simulink model "frequency_only"  (R2012b)
settings: Solver=ode45  StartTime=0.0  StopTime=41000*512  RelTol=1e-3
libraries: xbsIndex_r4 x14823, casper_library_misc x115, casper_library_multipliers x20, casper_library_delays x13, simulink x3, xps_library x3, dspsrcs4 x2, xbsReplacements_r4 x2
(part 5 of 146)

== system frequency_only/accumulators/accumulator_0x1 ==
  note: Note: in1 = MSB, in2 = LSB
  note: We want out vacc to keep full resolution
  new_acc : Inport
  bus_in : Inport  Port=2
  Convert{,1..3} (4 alike) : xbsIndex_r4/Convert  gui_display_data_type=Fixed-point  arith_type="Signed  (2's comp)"  n_bits=64  bin_pt=34  float_type=Single  exp_bits=8  fraction_bits=24  quantization=Truncate  overflow=Wrap  en=off  latency=0  dbl_ovrd=off  pipeline=off  block_type=convert
  Delay{,1..4} (5 alike) : xbsIndex_r4/Delay  rst=off  infoeditControl=Selection of Reset will increase slice count due to use of real FFs and instead of SRLs  en=off  latency=1  dbl_ovrd=off  reg_retiming=off  block_type=delay
  Logical : xbsIndex_r4/Logical  logical_function=OR  inputs=4  en=off  latency=1  precision=Full  arith_type=Unsigned  n_bits=16  bin_pt=0  align_bp=on  dbl_ovrd=off  block_type=logical
  Terminator : Terminator
  Terminator1 : Terminator
  Terminator2 : Terminator
  bus_create1 : Subsystem  AncestorBlock=casper_library_flow_control/bus_create  mask(bus_create){inputNum=2}
      mask prompts: inputNum "Number of inputs:"
      mask init:
      | bus_create_init(gcb,...
      |     'inputNum', inputNum);
  bus_create2 : Subsystem  AncestorBlock=casper_library_flow_control/bus_create  mask(bus_create){inputNum=2}
      mask prompts: inputNum "Number of inputs:"
      mask init:
      | bus_create_init(gcb,...
      |     'inputNum', inputNum);
  bus_create4 : Subsystem  AncestorBlock=casper_library_flow_control/bus_create  mask(bus_create){inputNum=2}
      mask prompts: inputNum "Number of inputs:"
      mask init:
      | bus_create_init(gcb,...
      |     'inputNum', inputNum);
  bus_expand : Subsystem  AncestorBlock=casper_library_flow_control/bus_expand  mask(bus_expand){mode=divisions of equal size, outputNum=2, outputWidth=bitwidth_in*2, outputBinaryPt=0, outputArithmeticType=0, show_format=off, outputToWorkspace=off, variablePrefix=out, outputToModelAsWell=on}
      mask prompts: outputNum "Number of outputs:"; outputWidth "Output width:"; outputBinaryPt "Output binary point position:"; outputArithmeticType "Output arithmetic type (ufix=0, fix=1, bool=2):"; show_format "Print format string?"; outputToWorkspace "Output to workspace?"; variablePrefix "Variable name prefix:"; outputToModelAsWell "Output to model as well?"
      mask help:
      | Expands a 'bus' made using a bus_create or Xilinx
      | concat block.
      | The input will be divided into the specified number
      | of outputs with the specified arithmetic types.
      | Divisions are made from most significant bit.
      mask init: same as frequency_only/bus_expand
      settings: AttributesFormatString=2 outputs
      mask TypeOptions mode: divisions of equal size | divisions of arbitrary size
      mask Callback mode: bus_expand_callback();
      mask Callback outputWidth: bus_expand_callback();
      mask Callback outputToWorkspace: bus_expand_callback();
  dsp48e_bram_vacc_lsb_im : Subsystem  AncestorBlock=casper_library_accumulators/dsp48e_bram_vacc  mask(dsp48e_bram_vacc){vec_len=vector_length, arith_type=Signed  (2's comp), bin_pt_in=bin_point_in, n_bits_out=bitwidth_out, convert_latency=1}
      mask prompts: vec_len "Vector length:"; arith_type "Output type:"; bin_pt_in "Binary point (input):"; n_bits_out "Bit width (output):"; convert_latency "Convert Latency"
      mask help:
      | A vector accumulator modeled after a shift register.  It outputs its previous accumulated vector after a new_acc pulse is received.
      |
      | Based on the simple_bram_vacc block, this version replaces the adder and mux with a single DSP48E block, allowing high-speed compilation.
      |
      | The input and outputs ports are limited to 48 bits. Overflow is indicated with a line out.
      |
      | Each accumulation uses the full 48 bits, irrespective of mask parameters.
      | The output of the accumulation then slices off the output bits.
      | The binary point is kept at the same relative location to ensure that the signal value is not changed.
      mask init:
      | dsp48e_bram_vacc_init(gcb, ...
      |     'vec_len', vec_len, ...
      |     'arith_type', arith_type, ...
      |     'bin_pt_in', bin_pt_in, ...
      |     'n_bits_out', n_bits_out, ...
      |     'convert_latency', convert_latency);
      mask TypeOptions arith_type: Unsigned | Signed  (2's comp)
  dsp48e_bram_vacc_lsb_re : Subsystem  AncestorBlock=casper_library_accumulators/dsp48e_bram_vacc  mask(dsp48e_bram_vacc){vec_len=vector_length, arith_type=Signed  (2's comp), bin_pt_in=bin_point_in, n_bits_out=bitwidth_out, convert_latency=1}
      mask prompts: vec_len "Vector length:"; arith_type "Output type:"; bin_pt_in "Binary point (input):"; n_bits_out "Bit width (output):"; convert_latency "Convert Latency"
      mask help:
      | A vector accumulator modeled after a shift register.  It outputs its previous accumulated vector after a new_acc pulse is received.
      |
      | Based on the simple_bram_vacc block, this version replaces the adder and mux with a single DSP48E block, allowing high-speed compilation.
      |
      | The input and outputs ports are limited to 48 bits. Overflow is indicated with a line out.
      |
      | Each accumulation uses the full 48 bits, irrespective of mask parameters.
      | The output of the accumulation then slices off the output bits.
      | The binary point is kept at the same relative location to ensure that the signal value is not changed.
      mask init:
      | dsp48e_bram_vacc_init(gcb, ...
      |     'vec_len', vec_len, ...
      |     'arith_type', arith_type, ...
      |     'bin_pt_in', bin_pt_in, ...
      |     'n_bits_out', n_bits_out, ...
      |     'convert_latency', convert_latency);
      mask TypeOptions arith_type: Unsigned | Signed  (2's comp)
  dsp48e_bram_vacc_msb_im : Subsystem  AncestorBlock=casper_library_accumulators/dsp48e_bram_vacc  mask(dsp48e_bram_vacc){vec_len=vector_length, arith_type=Signed  (2's comp), bin_pt_in=bin_point_in, n_bits_out=bitwidth_out, convert_latency=1}
      mask prompts: vec_len "Vector length:"; arith_type "Output type:"; bin_pt_in "Binary point (input):"; n_bits_out "Bit width (output):"; convert_latency "Convert Latency"
      mask help:
      | A vector accumulator modeled after a shift register.  It outputs its previous accumulated vector after a new_acc pulse is received.
      |
      | Based on the simple_bram_vacc block, this version replaces the adder and mux with a single DSP48E block, allowing high-speed compilation.
      |
      | The input and outputs ports are limited to 48 bits. Overflow is indicated with a line out.
      |
      | Each accumulation uses the full 48 bits, irrespective of mask parameters.
      | The output of the accumulation then slices off the output bits.
      | The binary point is kept at the same relative location to ensure that the signal value is not changed.
      mask init:
      | dsp48e_bram_vacc_init(gcb, ...
      |     'vec_len', vec_len, ...
      |     'arith_type', arith_type, ...
      |     'bin_pt_in', bin_pt_in, ...
      |     'n_bits_out', n_bits_out, ...
      |     'convert_latency', convert_latency);
      mask TypeOptions arith_type: Unsigned | Signed  (2's comp)
  dsp48e_bram_vacc_msb_re : Subsystem  AncestorBlock=casper_library_accumulators/dsp48e_bram_vacc  mask(dsp48e_bram_vacc){vec_len=vector_length, arith_type=Signed  (2's comp), bin_pt_in=bin_point_in, n_bits_out=bitwidth_out, convert_latency=1}
      mask prompts: vec_len "Vector length:"; arith_type "Output type:"; bin_pt_in "Binary point (input):"; n_bits_out "Bit width (output):"; convert_latency "Convert Latency"
      mask help:
      | A vector accumulator modeled after a shift register.  It outputs its previous accumulated vector after a new_acc pulse is received.
      |
      | Based on the simple_bram_vacc block, this version replaces the adder and mux with a single DSP48E block, allowing high-speed compilation.
      |
      | The input and outputs ports are limited to 48 bits. Overflow is indicated with a line out.
      |
      | Each accumulation uses the full 48 bits, irrespective of mask parameters.
      | The output of the accumulation then slices off the output bits.
      | The binary point is kept at the same relative location to ensure that the signal value is not changed.
      mask init:
      | dsp48e_bram_vacc_init(gcb, ...
      |     'vec_len', vec_len, ...
      |     'arith_type', arith_type, ...
      |     'bin_pt_in', bin_pt_in, ...
      |     'n_bits_out', n_bits_out, ...
      |     'convert_latency', convert_latency);
      mask TypeOptions arith_type: Unsigned | Signed  (2's comp)
  lsb_c_to_ri : casper_library_misc/c_to_ri  n_bits=bitwidth_in  bin_pt=bin_point_in
      settings: AttributesFormatString=37_34 r/i
  msb_c_to_ri : casper_library_misc/c_to_ri  n_bits=bitwidth_in  bin_pt=bin_point_in
      settings: AttributesFormatString=37_34 r/i
  acc_valid : Outport
  bus_out : Outport  Port=2
  carry : Outport  Port=3
  wires:
  Logical/1 -> carry/1
  [c_lsb_im] -> Logical/4
  [c_lsb_re] -> Logical/3
  [c_msb_im] -> Logical/2
  [c_msb_re] -> Logical/1
  dsp48e_bram_vacc_lsb_im/3(carry) -> [c_lsb_im]
  dsp48e_bram_vacc_lsb_im/1(dout) -> Convert3/1
  dsp48e_bram_vacc_lsb_re/3(carry) -> [c_lsb_re]
  dsp48e_bram_vacc_msb_im/3(carry) -> [c_msb_im]
  dsp48e_bram_vacc_msb_re/3(carry) -> [c_msb_re]
  Convert3/1 -> bus_create1/2(in2)
  Convert2/1 -> bus_create1/1(in1)
  Convert1/1 -> bus_create4/2(in2)
  Convert/1 -> bus_create4/1(in1)
  Delay4/1 -> dsp48e_bram_vacc_lsb_im/2(din)
  Delay3/1 -> dsp48e_bram_vacc_lsb_re/2(din)
  Delay2/1 -> dsp48e_bram_vacc_msb_im/2(din)
  Delay1/1 -> dsp48e_bram_vacc_msb_re/2(din)
  Delay/1 -> [new_acc]
  [new_acc] -> dsp48e_bram_vacc_msb_re/1(new_acc)
  lsb_c_to_ri/2 -> Delay4/1
  lsb_c_to_ri/1 -> Delay3/1
  msb_c_to_ri/2 -> Delay2/1
  msb_c_to_ri/1 -> Delay1/1
  bus_in/1 -> bus_expand/1(bus_in)
  bus_create2/1(bus_out) -> bus_out/1
  dsp48e_bram_vacc_msb_re/1(dout) -> Convert/1
  dsp48e_bram_vacc_msb_im/1(dout) -> Convert1/1
  dsp48e_bram_vacc_lsb_re/1(dout) -> Convert2/1
  new_acc/1 -> Delay/1
  bus_create1/1(bus_out) -> bus_create2/2(in2)
  bus_create4/1(bus_out) -> bus_create2/1(in1)
  [new_acc] -> dsp48e_bram_vacc_lsb_im/1(new_acc)
  [new_acc] -> dsp48e_bram_vacc_lsb_re/1(new_acc)
  [new_acc] -> dsp48e_bram_vacc_msb_im/1(new_acc)
  dsp48e_bram_vacc_msb_re/2(valid) -> acc_valid/1
  bus_expand/2(lsb_out1) -> lsb_c_to_ri/1
  bus_expand/1(msb_out2) -> msb_c_to_ri/1
  dsp48e_bram_vacc_lsb_re/2(valid) -> Terminator1/1
  dsp48e_bram_vacc_msb_im/2(valid) -> Terminator/1
  dsp48e_bram_vacc_lsb_im/2(valid) -> Terminator2/1

== system frequency_only/accumulators/accumulator_0x2 ==
  note: We want out vacc to keep full resolution
  note: Note: in1 = MSB, in2 = LSB
  new_acc : Inport
  bus_in : Inport  Port=2
  Convert{,1..3} (4 alike) : xbsIndex_r4/Convert  gui_display_data_type=Fixed-point  arith_type="Signed  (2's comp)"  n_bits=64  bin_pt=34  float_type=Single  exp_bits=8  fraction_bits=24  quantization=Truncate  overflow=Wrap  en=off  latency=0  dbl_ovrd=off  pipeline=off  block_type=convert
  Delay{,1..4} (5 alike) : xbsIndex_r4/Delay  rst=off  infoeditControl=Selection of Reset will increase slice count due to use of real FFs and instead of SRLs  en=off  latency=1  dbl_ovrd=off  reg_retiming=off  block_type=delay
  Logical : xbsIndex_r4/Logical  logical_function=OR  inputs=4  en=off  latency=1  precision=Full  arith_type=Unsigned  n_bits=16  bin_pt=0  align_bp=on  dbl_ovrd=off  block_type=logical
  Terminator : Terminator
  Terminator1 : Terminator
  Terminator2 : Terminator
  bus_create1 : Subsystem  AncestorBlock=casper_library_flow_control/bus_create  mask(bus_create){inputNum=2}
      mask prompts: inputNum "Number of inputs:"
      mask init:
      | bus_create_init(gcb,...
      |     'inputNum', inputNum);
  bus_create2 : Subsystem  AncestorBlock=casper_library_flow_control/bus_create  mask(bus_create){inputNum=2}
      mask prompts: inputNum "Number of inputs:"
      mask init:
      | bus_create_init(gcb,...
      |     'inputNum', inputNum);
  bus_create4 : Subsystem  AncestorBlock=casper_library_flow_control/bus_create  mask(bus_create){inputNum=2}
      mask prompts: inputNum "Number of inputs:"
      mask init:
      | bus_create_init(gcb,...
      |     'inputNum', inputNum);
  bus_expand : Subsystem  AncestorBlock=casper_library_flow_control/bus_expand  mask(bus_expand){mode=divisions of equal size, outputNum=2, outputWidth=bitwidth_in*2, outputBinaryPt=0, outputArithmeticType=0, show_format=off, outputToWorkspace=off, variablePrefix=out, outputToModelAsWell=on}
      mask prompts: outputNum "Number of outputs:"; outputWidth "Output width:"; outputBinaryPt "Output binary point position:"; outputArithmeticType "Output arithmetic type (ufix=0, fix=1, bool=2):"; show_format "Print format string?"; outputToWorkspace "Output to workspace?"; variablePrefix "Variable name prefix:"; outputToModelAsWell "Output to model as well?"
      mask help:
      | Expands a 'bus' made using a bus_create or Xilinx
      | concat block.
      | The input will be divided into the specified number
      | of outputs with the specified arithmetic types.
      | Divisions are made from most significant bit.
      mask init: same as frequency_only/bus_expand
      settings: AttributesFormatString=2 outputs
      mask TypeOptions mode: divisions of equal size | divisions of arbitrary size
      mask Callback mode: bus_expand_callback();
      mask Callback outputWidth: bus_expand_callback();
      mask Callback outputToWorkspace: bus_expand_callback();
  dsp48e_bram_vacc_lsb_im : Subsystem  AncestorBlock=casper_library_accumulators/dsp48e_bram_vacc  mask(dsp48e_bram_vacc){vec_len=vector_length, arith_type=Signed  (2's comp), bin_pt_in=bin_point_in, n_bits_out=bitwidth_out, convert_latency=1}
      mask prompts: vec_len "Vector length:"; arith_type "Output type:"; bin_pt_in "Binary point (input):"; n_bits_out "Bit width (output):"; convert_latency "Convert Latency"
      mask help:
      | A vector accumulator modeled after a shift register.  It outputs its previous accumulated vector after a new_acc pulse is received.
      |
      | Based on the simple_bram_vacc block, this version replaces the adder and mux with a single DSP48E block, allowing high-speed compilation.
      |
      | The input and outputs ports are limited to 48 bits. Overflow is indicated with a line out.
      |
      | Each accumulation uses the full 48 bits, irrespective of mask parameters.
      | The output of the accumulation then slices off the output bits.
      | The binary point is kept at the same relative location to ensure that the signal value is not changed.
      mask init:
      | dsp48e_bram_vacc_init(gcb, ...
      |     'vec_len', vec_len, ...
      |     'arith_type', arith_type, ...
      |     'bin_pt_in', bin_pt_in, ...
      |     'n_bits_out', n_bits_out, ...
      |     'convert_latency', convert_latency);
      mask TypeOptions arith_type: Unsigned | Signed  (2's comp)
  dsp48e_bram_vacc_lsb_re : Subsystem  AncestorBlock=casper_library_accumulators/dsp48e_bram_vacc  mask(dsp48e_bram_vacc){vec_len=vector_length, arith_type=Signed  (2's comp), bin_pt_in=bin_point_in, n_bits_out=bitwidth_out, convert_latency=1}
      mask prompts: vec_len "Vector length:"; arith_type "Output type:"; bin_pt_in "Binary point (input):"; n_bits_out "Bit width (output):"; convert_latency "Convert Latency"
      mask help:
      | A vector accumulator modeled after a shift register.  It outputs its previous accumulated vector after a new_acc pulse is received.
      |
      | Based on the simple_bram_vacc block, this version replaces the adder and mux with a single DSP48E block, allowing high-speed compilation.
      |
      | The input and outputs ports are limited to 48 bits. Overflow is indicated with a line out.
      |
      | Each accumulation uses the full 48 bits, irrespective of mask parameters.
      | The output of the accumulation then slices off the output bits.
      | The binary point is kept at the same relative location to ensure that the signal value is not changed.
      mask init:
      | dsp48e_bram_vacc_init(gcb, ...
      |     'vec_len', vec_len, ...
      |     'arith_type', arith_type, ...
      |     'bin_pt_in', bin_pt_in, ...
      |     'n_bits_out', n_bits_out, ...
      |     'convert_latency', convert_latency);
      mask TypeOptions arith_type: Unsigned | Signed  (2's comp)
  dsp48e_bram_vacc_msb_im : Subsystem  AncestorBlock=casper_library_accumulators/dsp48e_bram_vacc  mask(dsp48e_bram_vacc){vec_len=vector_length, arith_type=Signed  (2's comp), bin_pt_in=bin_point_in, n_bits_out=bitwidth_out, convert_latency=1}
      mask prompts: vec_len "Vector length:"; arith_type "Output type:"; bin_pt_in "Binary point (input):"; n_bits_out "Bit width (output):"; convert_latency "Convert Latency"
      mask help:
      | A vector accumulator modeled after a shift register.  It outputs its previous accumulated vector after a new_acc pulse is received.
      |
      | Based on the simple_bram_vacc block, this version replaces the adder and mux with a single DSP48E block, allowing high-speed compilation.
      |
      | The input and outputs ports are limited to 48 bits. Overflow is indicated with a line out.
      |
      | Each accumulation uses the full 48 bits, irrespective of mask parameters.
      | The output of the accumulation then slices off the output bits.
      | The binary point is kept at the same relative location to ensure that the signal value is not changed.
      mask init:
      | dsp48e_bram_vacc_init(gcb, ...
      |     'vec_len', vec_len, ...
      |     'arith_type', arith_type, ...
      |     'bin_pt_in', bin_pt_in, ...
      |     'n_bits_out', n_bits_out, ...
      |     'convert_latency', convert_latency);
      mask TypeOptions arith_type: Unsigned | Signed  (2's comp)
  dsp48e_bram_vacc_msb_re : Subsystem  AncestorBlock=casper_library_accumulators/dsp48e_bram_vacc  mask(dsp48e_bram_vacc){vec_len=vector_length, arith_type=Signed  (2's comp), bin_pt_in=bin_point_in, n_bits_out=bitwidth_out, convert_latency=1}
      mask prompts: vec_len "Vector length:"; arith_type "Output type:"; bin_pt_in "Binary point (input):"; n_bits_out "Bit width (output):"; convert_latency "Convert Latency"
      mask help:
      | A vector accumulator modeled after a shift register.  It outputs its previous accumulated vector after a new_acc pulse is received.
      |
      | Based on the simple_bram_vacc block, this version replaces the adder and mux with a single DSP48E block, allowing high-speed compilation.
      |
      | The input and outputs ports are limited to 48 bits. Overflow is indicated with a line out.
      |
      | Each accumulation uses the full 48 bits, irrespective of mask parameters.
      | The output of the accumulation then slices off the output bits.
      | The binary point is kept at the same relative location to ensure that the signal value is not changed.
      mask init:
      | dsp48e_bram_vacc_init(gcb, ...
      |     'vec_len', vec_len, ...
      |     'arith_type', arith_type, ...
      |     'bin_pt_in', bin_pt_in, ...
      |     'n_bits_out', n_bits_out, ...
      |     'convert_latency', convert_latency);
      mask TypeOptions arith_type: Unsigned | Signed  (2's comp)
  lsb_c_to_ri : casper_library_misc/c_to_ri  n_bits=bitwidth_in  bin_pt=bin_point_in
      settings: AttributesFormatString=37_34 r/i
  msb_c_to_ri : casper_library_misc/c_to_ri  n_bits=bitwidth_in  bin_pt=bin_point_in
      settings: AttributesFormatString=37_34 r/i
  acc_valid : Outport
  bus_out : Outport  Port=2
  carry : Outport  Port=3
  wires:
  dsp48e_bram_vacc_lsb_im/2(valid) -> Terminator2/1
  dsp48e_bram_vacc_msb_im/2(valid) -> Terminator/1
  dsp48e_bram_vacc_lsb_re/2(valid) -> Terminator1/1
  bus_expand/1(msb_out2) -> msb_c_to_ri/1
  bus_expand/2(lsb_out1) -> lsb_c_to_ri/1
  dsp48e_bram_vacc_msb_re/2(valid) -> acc_valid/1
  [new_acc] -> dsp48e_bram_vacc_msb_im/1(new_acc)
  [new_acc] -> dsp48e_bram_vacc_lsb_re/1(new_acc)
  [new_acc] -> dsp48e_bram_vacc_lsb_im/1(new_acc)
  bus_create4/1(bus_out) -> bus_create2/1(in1)
  bus_create1/1(bus_out) -> bus_create2/2(in2)
  new_acc/1 -> Delay/1
  dsp48e_bram_vacc_lsb_re/1(dout) -> Convert2/1
  dsp48e_bram_vacc_msb_im/1(dout) -> Convert1/1
  dsp48e_bram_vacc_msb_re/1(dout) -> Convert/1
  bus_create2/1(bus_out) -> bus_out/1
  bus_in/1 -> bus_expand/1(bus_in)
  msb_c_to_ri/1 -> Delay1/1
  msb_c_to_ri/2 -> Delay2/1
  lsb_c_to_ri/1 -> Delay3/1
  lsb_c_to_ri/2 -> Delay4/1
  [new_acc] -> dsp48e_bram_vacc_msb_re/1(new_acc)
  Delay/1 -> [new_acc]
  Delay1/1 -> dsp48e_bram_vacc_msb_re/2(din)
  Delay2/1 -> dsp48e_bram_vacc_msb_im/2(din)
  Delay3/1 -> dsp48e_bram_vacc_lsb_re/2(din)
  Delay4/1 -> dsp48e_bram_vacc_lsb_im/2(din)
  Convert/1 -> bus_create4/1(in1)
  Convert1/1 -> bus_create4/2(in2)
  Convert2/1 -> bus_create1/1(in1)
  Convert3/1 -> bus_create1/2(in2)
  dsp48e_bram_vacc_msb_re/3(carry) -> [c_msb_re]
  dsp48e_bram_vacc_msb_im/3(carry) -> [c_msb_im]
  dsp48e_bram_vacc_lsb_re/3(carry) -> [c_lsb_re]
  dsp48e_bram_vacc_lsb_im/1(dout) -> Convert3/1
  dsp48e_bram_vacc_lsb_im/3(carry) -> [c_lsb_im]
  [c_msb_re] -> Logical/1
  [c_msb_im] -> Logical/2
  [c_lsb_re] -> Logical/3
  [c_lsb_im] -> Logical/4
  Logical/1 -> carry/1

== system frequency_only/accumulators/accumulator_0x3 ==
  note: Note: in1 = MSB, in2 = LSB
  note: We want out vacc to keep full resolution
  new_acc : Inport
  bus_in : Inport  Port=2
  Convert{,1..3} (4 alike) : xbsIndex_r4/Convert  gui_display_data_type=Fixed-point  arith_type="Signed  (2's comp)"  n_bits=64  bin_pt=34  float_type=Single  exp_bits=8  fraction_bits=24  quantization=Truncate  overflow=Wrap  en=off  latency=0  dbl_ovrd=off  pipeline=off  block_type=convert
  Delay{,1..4} (5 alike) : xbsIndex_r4/Delay  rst=off  infoeditControl=Selection of Reset will increase slice count due to use of real FFs and instead of SRLs  en=off  latency=1  dbl_ovrd=off  reg_retiming=off  block_type=delay
  Logical : xbsIndex_r4/Logical  logical_function=OR  inputs=4  en=off  latency=1  precision=Full  arith_type=Unsigned  n_bits=16  bin_pt=0  align_bp=on  dbl_ovrd=off  block_type=logical
  Terminator : Terminator
  Terminator1 : Terminator
  Terminator2 : Terminator
  bus_create1 : Subsystem  AncestorBlock=casper_library_flow_control/bus_create  mask(bus_create){inputNum=2}
      mask prompts: inputNum "Number of inputs:"
      mask init:
      | bus_create_init(gcb,...
      |     'inputNum', inputNum);
  bus_create2 : Subsystem  AncestorBlock=casper_library_flow_control/bus_create  mask(bus_create){inputNum=2}
      mask prompts: inputNum "Number of inputs:"
      mask init:
      | bus_create_init(gcb,...
      |     'inputNum', inputNum);
  bus_create4 : Subsystem  AncestorBlock=casper_library_flow_control/bus_create  mask(bus_create){inputNum=2}
      mask prompts: inputNum "Number of inputs:"
      mask init:
      | bus_create_init(gcb,...
      |     'inputNum', inputNum);
  bus_expand : Subsystem  AncestorBlock=casper_library_flow_control/bus_expand  mask(bus_expand){mode=divisions of equal size, outputNum=2, outputWidth=bitwidth_in*2, outputBinaryPt=0, outputArithmeticType=0, show_format=off, outputToWorkspace=off, variablePrefix=out, outputToModelAsWell=on}
      mask prompts: outputNum "Number of outputs:"; outputWidth "Output width:"; outputBinaryPt "Output binary point position:"; outputArithmeticType "Output arithmetic type (ufix=0, fix=1, bool=2):"; show_format "Print format string?"; outputToWorkspace "Output to workspace?"; variablePrefix "Variable name prefix:"; outputToModelAsWell "Output to model as well?"
      mask help:
      | Expands a 'bus' made using a bus_create or Xilinx
      | concat block.
      | The input will be divided into the specified number
      | of outputs with the specified arithmetic types.
      | Divisions are made from most significant bit.
      mask init: same as frequency_only/bus_expand
      settings: AttributesFormatString=2 outputs
      mask TypeOptions mode: divisions of equal size | divisions of arbitrary size
      mask Callback mode: bus_expand_callback();
      mask Callback outputWidth: bus_expand_callback();
      mask Callback outputToWorkspace: bus_expand_callback();
  dsp48e_bram_vacc_lsb_im : Subsystem  AncestorBlock=casper_library_accumulators/dsp48e_bram_vacc  mask(dsp48e_bram_vacc){vec_len=vector_length, arith_type=Signed  (2's comp), bin_pt_in=bin_point_in, n_bits_out=bitwidth_out, convert_latency=1}
      mask prompts: vec_len "Vector length:"; arith_type "Output type:"; bin_pt_in "Binary point (input):"; n_bits_out "Bit width (output):"; convert_latency "Convert Latency"
      mask help:
      | A vector accumulator modeled after a shift register.  It outputs its previous accumulated vector after a new_acc pulse is received.
      |
      | Based on the simple_bram_vacc block, this version replaces the adder and mux with a single DSP48E block, allowing high-speed compilation.
      |
      | The input and outputs ports are limited to 48 bits. Overflow is indicated with a line out.
      |
      | Each accumulation uses the full 48 bits, irrespective of mask parameters.
      | The output of the accumulation then slices off the output bits.
      | The binary point is kept at the same relative location to ensure that the signal value is not changed.
      mask init:
      | dsp48e_bram_vacc_init(gcb, ...
      |     'vec_len', vec_len, ...
      |     'arith_type', arith_type, ...
      |     'bin_pt_in', bin_pt_in, ...
      |     'n_bits_out', n_bits_out, ...
      |     'convert_latency', convert_latency);
      mask TypeOptions arith_type: Unsigned | Signed  (2's comp)
  dsp48e_bram_vacc_lsb_re : Subsystem  AncestorBlock=casper_library_accumulators/dsp48e_bram_vacc  mask(dsp48e_bram_vacc){vec_len=vector_length, arith_type=Signed  (2's comp), bin_pt_in=bin_point_in, n_bits_out=bitwidth_out, convert_latency=1}
      mask prompts: vec_len "Vector length:"; arith_type "Output type:"; bin_pt_in "Binary point (input):"; n_bits_out "Bit width (output):"; convert_latency "Convert Latency"
      mask help:
      | A vector accumulator modeled after a shift register.  It outputs its previous accumulated vector after a new_acc pulse is received.
      |
      | Based on the simple_bram_vacc block, this version replaces the adder and mux with a single DSP48E block, allowing high-speed compilation.
      |
      | The input and outputs ports are limited to 48 bits. Overflow is indicated with a line out.
      |
      | Each accumulation uses the full 48 bits, irrespective of mask parameters.
      | The output of the accumulation then slices off the output bits.
      | The binary point is kept at the same relative location to ensure that the signal value is not changed.
      mask init:
      | dsp48e_bram_vacc_init(gcb, ...
      |     'vec_len', vec_len, ...
      |     'arith_type', arith_type, ...
      |     'bin_pt_in', bin_pt_in, ...
      |     'n_bits_out', n_bits_out, ...
      |     'convert_latency', convert_latency);
      mask TypeOptions arith_type: Unsigned | Signed  (2's comp)
  dsp48e_bram_vacc_msb_im : Subsystem  AncestorBlock=casper_library_accumulators/dsp48e_bram_vacc  mask(dsp48e_bram_vacc){vec_len=vector_length, arith_type=Signed  (2's comp), bin_pt_in=bin_point_in, n_bits_out=bitwidth_out, convert_latency=1}
      mask prompts: vec_len "Vector length:"; arith_type "Output type:"; bin_pt_in "Binary point (input):"; n_bits_out "Bit width (output):"; convert_latency "Convert Latency"
      mask help:
      | A vector accumulator modeled after a shift register.  It outputs its previous accumulated vector after a new_acc pulse is received.
      |
      | Based on the simple_bram_vacc block, this version replaces the adder and mux with a single DSP48E block, allowing high-speed compilation.
      |
      | The input and outputs ports are limited to 48 bits. Overflow is indicated with a line out.
      |
      | Each accumulation uses the full 48 bits, irrespective of mask parameters.
      | The output of the accumulation then slices off the output bits.
      | The binary point is kept at the same relative location to ensure that the signal value is not changed.
      mask init:
      | dsp48e_bram_vacc_init(gcb, ...
      |     'vec_len', vec_len, ...
      |     'arith_type', arith_type, ...
      |     'bin_pt_in', bin_pt_in, ...
      |     'n_bits_out', n_bits_out, ...
      |     'convert_latency', convert_latency);
      mask TypeOptions arith_type: Unsigned | Signed  (2's comp)
  dsp48e_bram_vacc_msb_re : Subsystem  AncestorBlock=casper_library_accumulators/dsp48e_bram_vacc  mask(dsp48e_bram_vacc){vec_len=vector_length, arith_type=Signed  (2's comp), bin_pt_in=bin_point_in, n_bits_out=bitwidth_out, convert_latency=1}
      mask prompts: vec_len "Vector length:"; arith_type "Output type:"; bin_pt_in "Binary point (input):"; n_bits_out "Bit width (output):"; convert_latency "Convert Latency"
      mask help:
      | A vector accumulator modeled after a shift register.  It outputs its previous accumulated vector after a new_acc pulse is received.
      |
      | Based on the simple_bram_vacc block, this version replaces the adder and mux with a single DSP48E block, allowing high-speed compilation.
      |
      | The input and outputs ports are limited to 48 bits. Overflow is indicated with a line out.
      |
      | Each accumulation uses the full 48 bits, irrespective of mask parameters.
      | The output of the accumulation then slices off the output bits.
      | The binary point is kept at the same relative location to ensure that the signal value is not changed.
      mask init:
      | dsp48e_bram_vacc_init(gcb, ...
      |     'vec_len', vec_len, ...
      |     'arith_type', arith_type, ...
      |     'bin_pt_in', bin_pt_in, ...
      |     'n_bits_out', n_bits_out, ...
      |     'convert_latency', convert_latency);
      mask TypeOptions arith_type: Unsigned | Signed  (2's comp)
  lsb_c_to_ri : casper_library_misc/c_to_ri  n_bits=bitwidth_in  bin_pt=bin_point_in
      settings: AttributesFormatString=37_34 r/i
  msb_c_to_ri : casper_library_misc/c_to_ri  n_bits=bitwidth_in  bin_pt=bin_point_in
      settings: AttributesFormatString=37_34 r/i
  acc_valid : Outport
  bus_out : Outport  Port=2
  carry : Outport  Port=3
  wires:
  Logical/1 -> carry/1
  [c_lsb_im] -> Logical/4
  [c_lsb_re] -> Logical/3
  [c_msb_im] -> Logical/2
  [c_msb_re] -> Logical/1
  dsp48e_bram_vacc_lsb_im/3(carry) -> [c_lsb_im]
  dsp48e_bram_vacc_lsb_im/1(dout) -> Convert3/1
  dsp48e_bram_vacc_lsb_re/3(carry) -> [c_lsb_re]
  dsp48e_bram_vacc_msb_im/3(carry) -> [c_msb_im]
  dsp48e_bram_vacc_msb_re/3(carry) -> [c_msb_re]
  Convert3/1 -> bus_create1/2(in2)
  Convert2/1 -> bus_create1/1(in1)
  Convert1/1 -> bus_create4/2(in2)
  Convert/1 -> bus_create4/1(in1)
  Delay4/1 -> dsp48e_bram_vacc_lsb_im/2(din)
  Delay3/1 -> dsp48e_bram_vacc_lsb_re/2(din)
  Delay2/1 -> dsp48e_bram_vacc_msb_im/2(din)
  Delay1/1 -> dsp48e_bram_vacc_msb_re/2(din)
  Delay/1 -> [new_acc]
  [new_acc] -> dsp48e_bram_vacc_msb_re/1(new_acc)
  lsb_c_to_ri/2 -> Delay4/1
  lsb_c_to_ri/1 -> Delay3/1
  msb_c_to_ri/2 -> Delay2/1
  msb_c_to_ri/1 -> Delay1/1
  bus_in/1 -> bus_expand/1(bus_in)
  bus_create2/1(bus_out) -> bus_out/1
  dsp48e_bram_vacc_msb_re/1(dout) -> Convert/1
  dsp48e_bram_vacc_msb_im/1(dout) -> Convert1/1
  dsp48e_bram_vacc_lsb_re/1(dout) -> Convert2/1
  new_acc/1 -> Delay/1
  bus_create1/1(bus_out) -> bus_create2/2(in2)
  bus_create4/1(bus_out) -> bus_create2/1(in1)
  [new_acc] -> dsp48e_bram_vacc_lsb_im/1(new_acc)
  [new_acc] -> dsp48e_bram_vacc_lsb_re/1(new_acc)
  [new_acc] -> dsp48e_bram_vacc_msb_im/1(new_acc)
  dsp48e_bram_vacc_msb_re/2(valid) -> acc_valid/1
  bus_expand/2(lsb_out1) -> lsb_c_to_ri/1
  bus_expand/1(msb_out2) -> msb_c_to_ri/1
  dsp48e_bram_vacc_lsb_re/2(valid) -> Terminator1/1
  dsp48e_bram_vacc_msb_im/2(valid) -> Terminator/1
  dsp48e_bram_vacc_lsb_im/2(valid) -> Terminator2/1

== system frequency_only/accumulators/accumulator_1x2 ==
  note: We want out vacc to keep full resolution
  note: Note: in1 = MSB, in2 = LSB
  new_acc : Inport
  bus_in : Inport  Port=2
  Convert{,1..3} (4 alike) : xbsIndex_r4/Convert  gui_display_data_type=Fixed-point  arith_type="Signed  (2's comp)"  n_bits=64  bin_pt=34  float_type=Single  exp_bits=8  fraction_bits=24  quantization=Truncate  overflow=Wrap  en=off  latency=0  dbl_ovrd=off  pipeline=off  block_type=convert
  Delay{,1..4} (5 alike) : xbsIndex_r4/Delay  rst=off  infoeditControl=Selection of Reset will increase slice count due to use of real FFs and instead of SRLs  en=off  latency=1  dbl_ovrd=off  reg_retiming=off  block_type=delay
  Logical : xbsIndex_r4/Logical  logical_function=OR  inputs=4  en=off  latency=1  precision=Full  arith_type=Unsigned  n_bits=16  bin_pt=0  align_bp=on  dbl_ovrd=off  block_type=logical
  Terminator : Terminator
  Terminator1 : Terminator
  Terminator2 : Terminator
  bus_create1 : Subsystem  AncestorBlock=casper_library_flow_control/bus_create  mask(bus_create){inputNum=2}
      mask prompts: inputNum "Number of inputs:"
      mask init:
      | bus_create_init(gcb,...
      |     'inputNum', inputNum);
  bus_create2 : Subsystem  AncestorBlock=casper_library_flow_control/bus_create  mask(bus_create){inputNum=2}
      mask prompts: inputNum "Number of inputs:"
      mask init:
      | bus_create_init(gcb,...
      |     'inputNum', inputNum);
  bus_create4 : Subsystem  AncestorBlock=casper_library_flow_control/bus_create  mask(bus_create){inputNum=2}
      mask prompts: inputNum "Number of inputs:"
      mask init:
      | bus_create_init(gcb,...
      |     'inputNum', inputNum);
  bus_expand : Subsystem  AncestorBlock=casper_library_flow_control/bus_expand  mask(bus_expand){mode=divisions of equal size, outputNum=2, outputWidth=bitwidth_in*2, outputBinaryPt=0, outputArithmeticType=0, show_format=off, outputToWorkspace=off, variablePrefix=out, outputToModelAsWell=on}
      mask prompts: outputNum "Number of outputs:"; outputWidth "Output width:"; outputBinaryPt "Output binary point position:"; outputArithmeticType "Output arithmetic type (ufix=0, fix=1, bool=2):"; show_format "Print format string?"; outputToWorkspace "Output to workspace?"; variablePrefix "Variable name prefix:"; outputToModelAsWell "Output to model as well?"
      mask help:
      | Expands a 'bus' made using a bus_create or Xilinx
      | concat block.
      | The input will be divided into the specified number
      | of outputs with the specified arithmetic types.
      | Divisions are made from most significant bit.
      mask init: same as frequency_only/bus_expand
      settings: AttributesFormatString=2 outputs
      mask TypeOptions mode: divisions of equal size | divisions of arbitrary size
      mask Callback mode: bus_expand_callback();
      mask Callback outputWidth: bus_expand_callback();
      mask Callback outputToWorkspace: bus_expand_callback();
  dsp48e_bram_vacc_lsb_im : Subsystem  AncestorBlock=casper_library_accumulators/dsp48e_bram_vacc  mask(dsp48e_bram_vacc){vec_len=vector_length, arith_type=Signed  (2's comp), bin_pt_in=bin_point_in, n_bits_out=bitwidth_out, convert_latency=1}
      mask prompts: vec_len "Vector length:"; arith_type "Output type:"; bin_pt_in "Binary point (input):"; n_bits_out "Bit width (output):"; convert_latency "Convert Latency"
      mask help:
      | A vector accumulator modeled after a shift register.  It outputs its previous accumulated vector after a new_acc pulse is received.
      |
      | Based on the simple_bram_vacc block, this version replaces the adder and mux with a single DSP48E block, allowing high-speed compilation.
      |
      | The input and outputs ports are limited to 48 bits. Overflow is indicated with a line out.
      |
      | Each accumulation uses the full 48 bits, irrespective of mask parameters.
      | The output of the accumulation then slices off the output bits.
      | The binary point is kept at the same relative location to ensure that the signal value is not changed.
      mask init:
      | dsp48e_bram_vacc_init(gcb, ...
      |     'vec_len', vec_len, ...
      |     'arith_type', arith_type, ...
      |     'bin_pt_in', bin_pt_in, ...
      |     'n_bits_out', n_bits_out, ...
      |     'convert_latency', convert_latency);
      mask TypeOptions arith_type: Unsigned | Signed  (2's comp)
  dsp48e_bram_vacc_lsb_re : Subsystem  AncestorBlock=casper_library_accumulators/dsp48e_bram_vacc  mask(dsp48e_bram_vacc){vec_len=vector_length, arith_type=Signed  (2's comp), bin_pt_in=bin_point_in, n_bits_out=bitwidth_out, convert_latency=1}
      mask prompts: vec_len "Vector length:"; arith_type "Output type:"; bin_pt_in "Binary point (input):"; n_bits_out "Bit width (output):"; convert_latency "Convert Latency"
      mask help:
      | A vector accumulator modeled after a shift register.  It outputs its previous accumulated vector after a new_acc pulse is received.
      |
      | Based on the simple_bram_vacc block, this version replaces the adder and mux with a single DSP48E block, allowing high-speed compilation.
      |
      | The input and outputs ports are limited to 48 bits. Overflow is indicated with a line out.
      |
      | Each accumulation uses the full 48 bits, irrespective of mask parameters.
      | The output of the accumulation then slices off the output bits.
      | The binary point is kept at the same relative location to ensure that the signal value is not changed.
      mask init:
      | dsp48e_bram_vacc_init(gcb, ...
      |     'vec_len', vec_len, ...
      |     'arith_type', arith_type, ...
      |     'bin_pt_in', bin_pt_in, ...
      |     'n_bits_out', n_bits_out, ...
      |     'convert_latency', convert_latency);
      mask TypeOptions arith_type: Unsigned | Signed  (2's comp)
  dsp48e_bram_vacc_msb_im : Subsystem  AncestorBlock=casper_library_accumulators/dsp48e_bram_vacc  mask(dsp48e_bram_vacc){vec_len=vector_length, arith_type=Signed  (2's comp), bin_pt_in=bin_point_in, n_bits_out=bitwidth_out, convert_latency=1}
      mask prompts: vec_len "Vector length:"; arith_type "Output type:"; bin_pt_in "Binary point (input):"; n_bits_out "Bit width (output):"; convert_latency "Convert Latency"
      mask help:
      | A vector accumulator modeled after a shift register.  It outputs its previous accumulated vector after a new_acc pulse is received.
      |
      | Based on the simple_bram_vacc block, this version replaces the adder and mux with a single DSP48E block, allowing high-speed compilation.
      |
      | The input and outputs ports are limited to 48 bits. Overflow is indicated with a line out.
      |
      | Each accumulation uses the full 48 bits, irrespective of mask parameters.
      | The output of the accumulation then slices off the output bits.
      | The binary point is kept at the same relative location to ensure that the signal value is not changed.
      mask init:
      | dsp48e_bram_vacc_init(gcb, ...
      |     'vec_len', vec_len, ...
      |     'arith_type', arith_type, ...
      |     'bin_pt_in', bin_pt_in, ...
      |     'n_bits_out', n_bits_out, ...
      |     'convert_latency', convert_latency);
      mask TypeOptions arith_type: Unsigned | Signed  (2's comp)
  dsp48e_bram_vacc_msb_re : Subsystem  AncestorBlock=casper_library_accumulators/dsp48e_bram_vacc  mask(dsp48e_bram_vacc){vec_len=vector_length, arith_type=Signed  (2's comp), bin_pt_in=bin_point_in, n_bits_out=bitwidth_out, convert_latency=1}
      mask prompts: vec_len "Vector length:"; arith_type "Output type:"; bin_pt_in "Binary point (input):"; n_bits_out "Bit width (output):"; convert_latency "Convert Latency"
      mask help:
      | A vector accumulator modeled after a shift register.  It outputs its previous accumulated vector after a new_acc pulse is received.
      |
      | Based on the simple_bram_vacc block, this version replaces the adder and mux with a single DSP48E block, allowing high-speed compilation.
      |
      | The input and outputs ports are limited to 48 bits. Overflow is indicated with a line out.
      |
      | Each accumulation uses the full 48 bits, irrespective of mask parameters.
      | The output of the accumulation then slices off the output bits.
      | The binary point is kept at the same relative location to ensure that the signal value is not changed.
      mask init:
      | dsp48e_bram_vacc_init(gcb, ...
      |     'vec_len', vec_len, ...
      |     'arith_type', arith_type, ...
      |     'bin_pt_in', bin_pt_in, ...
      |     'n_bits_out', n_bits_out, ...
      |     'convert_latency', convert_latency);
      mask TypeOptions arith_type: Unsigned | Signed  (2's comp)
  lsb_c_to_ri : casper_library_misc/c_to_ri  n_bits=bitwidth_in  bin_pt=bin_point_in
      settings: AttributesFormatString=37_34 r/i
  msb_c_to_ri : casper_library_misc/c_to_ri  n_bits=bitwidth_in  bin_pt=bin_point_in
      settings: AttributesFormatString=37_34 r/i
  acc_valid : Outport
  bus_out : Outport  Port=2
  carry : Outport  Port=3
  wires:
  dsp48e_bram_vacc_lsb_im/2(valid) -> Terminator2/1
  dsp48e_bram_vacc_msb_im/2(valid) -> Terminator/1
  dsp48e_bram_vacc_lsb_re/2(valid) -> Terminator1/1
  bus_expand/1(msb_out2) -> msb_c_to_ri/1
  bus_expand/2(lsb_out1) -> lsb_c_to_ri/1
  dsp48e_bram_vacc_msb_re/2(valid) -> acc_valid/1
  [new_acc] -> dsp48e_bram_vacc_msb_im/1(new_acc)
  [new_acc] -> dsp48e_bram_vacc_lsb_re/1(new_acc)
  [new_acc] -> dsp48e_bram_vacc_lsb_im/1(new_acc)
  bus_create4/1(bus_out) -> bus_create2/1(in1)
  bus_create1/1(bus_out) -> bus_create2/2(in2)
  new_acc/1 -> Delay/1
  dsp48e_bram_vacc_lsb_re/1(dout) -> Convert2/1
  dsp48e_bram_vacc_msb_im/1(dout) -> Convert1/1
  dsp48e_bram_vacc_msb_re/1(dout) -> Convert/1
  bus_create2/1(bus_out) -> bus_out/1
  bus_in/1 -> bus_expand/1(bus_in)
  msb_c_to_ri/1 -> Delay1/1
  msb_c_to_ri/2 -> Delay2/1
  lsb_c_to_ri/1 -> Delay3/1
  lsb_c_to_ri/2 -> Delay4/1
  [new_acc] -> dsp48e_bram_vacc_msb_re/1(new_acc)
  Delay/1 -> [new_acc]
  Delay1/1 -> dsp48e_bram_vacc_msb_re/2(din)
  Delay2/1 -> dsp48e_bram_vacc_msb_im/2(din)
  Delay3/1 -> dsp48e_bram_vacc_lsb_re/2(din)
  Delay4/1 -> dsp48e_bram_vacc_lsb_im/2(din)
  Convert/1 -> bus_create4/1(in1)
  Convert1/1 -> bus_create4/2(in2)
  Convert2/1 -> bus_create1/1(in1)
  Convert3/1 -> bus_create1/2(in2)
  dsp48e_bram_vacc_msb_re/3(carry) -> [c_msb_re]
  dsp48e_bram_vacc_msb_im/3(carry) -> [c_msb_im]
  dsp48e_bram_vacc_lsb_re/3(carry) -> [c_lsb_re]
  dsp48e_bram_vacc_lsb_im/1(dout) -> Convert3/1
  dsp48e_bram_vacc_lsb_im/3(carry) -> [c_lsb_im]
  [c_msb_re] -> Logical/1
  [c_msb_im] -> Logical/2
  [c_lsb_re] -> Logical/3
  [c_lsb_im] -> Logical/4
  Logical/1 -> carry/1
